simulink model "feed_fwd_2"  (Simulink 7.4)
settings: Solver=ode45  StartTime=0.0  StopTime=16e-6  MaxStep=1/(11*2140e6)  RelTol=1e-3
undefined symbols (not defined in the file): Fs, sided, Two
libraries: dsparch4 x10, dspsnks4 x3, simulink x1
settings Model: Creator=Dick  LastModifiedBy=Dick
settings DataIOCC: SignalLoggingName=sigsOut
settings OptimizationCC: BooleanDataType=off  InlineInvariantSignals=on  InitFltsAndDblsToZero=on
settings DebuggingCC: SaveWithParameterizedLinksMsg=none  SignalResolutionControl=TryResolveAllWithWarning  SolverPrmCheckMsg=none  MultiTaskDSMMsg=warning  MultiTaskCondExecSysMsg=none  StrictBusMsg=None
settings HardwareCC: TargetUnknown=on
settings RTWCC: IncludeERTFirstTime=on
settings GRTTargetCC: TargetFcnLib=ansi_tfl_tmw.mat

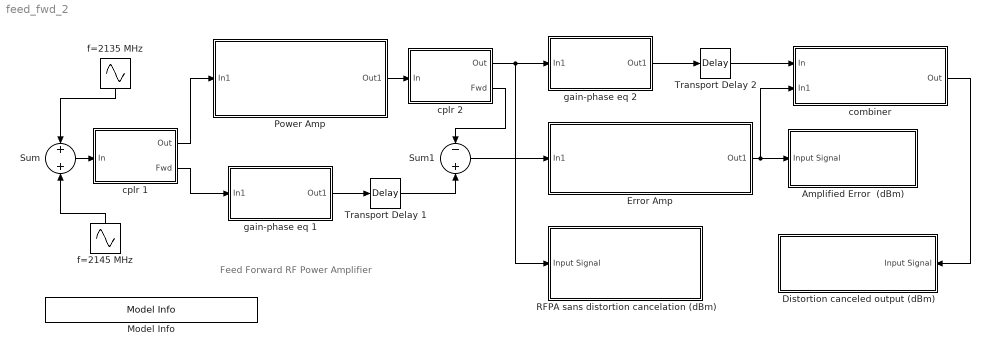
== system feed_fwd_2 ==
  note: Feed Forward RF Power Amplifier
  "  cplr 1" : Subsystem  mask{cplfac=-10}
      mask prompts: cplfac "Coupling Factor (in dB) ="
      mask Display: fprintf('Coupler  \n %5.2f dB', cplfac)
  "  cplr 2" : Subsystem  mask{cplfac=-6}
      mask prompts: cplfac "Coupling Factor (in dB) ="
      mask Display: disp(sprintf('Coupler  \n %5.2f dB', cplfac))
  Amplified Error  (dBm) : Subsystem  Description=Spectrum Analyzer  mask{BW=100e6, Fc=2140e6}
      mask prompts: BW "Bandwidth"; Fc "Center Freq"
      mask Display: fprintf('Spectrum Analyzer \n Fc=%7.2f MHz \n BW=%7.2f MHz',Fc/1e6,BW/1e6)
  Distortion canceled output (dBm) : Subsystem  Description=Spectrum Analyzer  mask{BW=100e6, Fc=2140e6}
      mask prompts: BW "Bandwidth"; Fc "Center Freq"
      mask Display: fprintf('Spectrum Analyzer \n Fc=%7.2f MHz \n BW=%7.2f MHz',Fc/1e6,BW/1e6)
  Error Amp : Subsystem  mask{dbg=12, Fc=2140, BW=100, Td=2}
      mask prompts: dbg "Gain in dB:"; Fc "Fcenter (MHz):"; BW "BW (MHz):"; Td "Time Delay (ns) :"
      mask Display:
      | fprintf(' Error Amp   Pg = %5.0f dB\n\n\n ',dbg);
      | fprintf(' Fcenter= %8.0f      BW= %5.0f MHz ', Fc, BW);
      | fprintf('\n\n\nTime Delay =%9.2f ns', Td);
  Model Info : simulink/Model-Wide Utilities/Model Info  SystemSampleTime=-1  InitialBlockCM=None  BlockCM=None  Frame=on  DisplayStringWithTags=Copywrite 2005-2010 The MathWorks, Inc.  HorizontalTextAlignment=Center  LeftAlignmentValue=0.5  SourceBlockDiagram=feed_fwd_2  TagMaxNumber=20
  Power Amp : Subsystem  mask{dbg=20, Fc=2140, BW=100, alpha=.02, Td=5}
      mask prompts: dbg "Gain in dB:"; Fc "Fcenter (MHz):"; BW "BW (MHz):"; alpha "Nonlinearity (0-1) :"; Td "Time Delay (ns) :"
      mask Display:
      | fprintf(' RFPA     Pg = %5.0f dB\n\n\n ',dbg);
      | fprintf('Fc= %6.0f    BW= %4.0fMHz ', Fc,BW);
      | fprintf('\n\n Nonlinearity =%9.4f', alpha);
      | fprintf('\n\n\n\n Time Delay =%9.2f ns', Td);
  RFPA sans distortion cancelation (dBm) : Subsystem  Description=Spectrum Analyzer  mask{BW=100e6, Fc=2140e6}
      mask prompts: BW "Bandwidth"; Fc "Center Freq"
      mask Display: fprintf('Spectrum Analyzer \n Fc=%7.2f MHz \n BW=%7.2f MHz',Fc/1e6,BW/1e6)
  Sum : Sum  OutDataType=sfix(16)  OutScaling=2^0  SaturateOnIntegerOverflow=on  InputSameDT=on  OutDataTypeStr=Inherit: Same as first input
  Sum1 : Sum  Inputs=-+  OutDataType=sfix(16)  OutScaling=2^0  SaturateOnIntegerOverflow=on  InputSameDT=on  OutDataTypeStr=Inherit: Same as first input
  Transport Delay 1 : TransportDelay  DelayTime=5e-9
  Transport Delay 2 : TransportDelay  DelayTime=2.0e-9
  combiner : Subsystem  mask{cplfac=-6}
      mask prompts: cplfac "Coupling Factor (in dB) ="
      mask Display: fprintf('Injection Coupler  \n %5.2f dB', cplfac)
  f=2135 MHz : Sin  Amplitude="((8e-3*50*10^(20/10))^0.5) /2    %  20 dBm"  Bias=0  Frequency=2*pi*(2140-5)*1e6;  Phase=0  Samples=10  SampleTime=0  Offset=0
  f=2145 MHz : Sin  Amplitude="((8e-3*50*10^(20/10))^0.5) /2    %  20 dBm"  Bias=0  Frequency=2*pi*(2140+5)*1e6  Phase=0  Samples=10  SampleTime=0  Offset=0
  gain-phase eq 1 : Subsystem
  gain-phase eq 2 : Subsystem
  wires:
  f=2135 MHz/1 -> Sum/1
  f=2145 MHz/1 -> Sum/2
  Sum/1 -> "  cplr 1"/1(In)
  "  cplr 1"/1(Out) -> Power Amp/1(In1)
  "  cplr 1"/2(Fwd) -> gain-phase eq 1/1(In1)
  gain-phase eq 1/1(Out1) -> Transport Delay 1/1
  Transport Delay 1/1 -> Sum1/2
  Sum1/1 -> Error Amp/1(In1)
  gain-phase eq 2/1(Out1) -> Transport Delay 2/1
  Transport Delay 2/1 -> combiner/1(In)
  Error Amp/1(Out1) -> combiner/2(In1), Amplified Error  (dBm)/1(Input Signal)
  combiner/1(Out) -> Distortion canceled output (dBm)/1(Input Signal)
  Power Amp/1(Out1) -> "  cplr 2"/1(In)
  "  cplr 2"/1(Out) -> gain-phase eq 2/1(In1), RFPA sans distortion cancelation (dBm)/1(Input Signal)
  "  cplr 2"/2(Fwd) -> Sum1/1

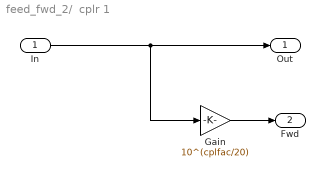
== system feed_fwd_2/  cplr 1 ==
  In : Inport  OutDataType=sfix(16)  OutScaling=2^0
  Gain : Gain  Gain=10^(cplfac/20)  ParameterDataType=sfix(16)  ParameterScaling=2^0  OutDataType=sfix(16)  OutScaling=2^0  SaturateOnIntegerOverflow=on  OutDataTypeStr=Inherit: Same as input  ParamDataTypeStr=Inherit: Same as input
  Out : Outport  OutDataType=sfix(16)  OutScaling=2^0
  Fwd : Outport  Port=2  OutDataType=sfix(16)  OutScaling=2^0
  wires:
  In/1 -> Out/1, Gain/1
  Gain/1 -> Fwd/1

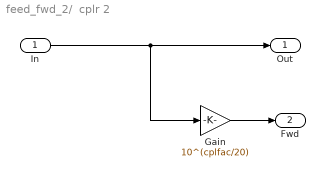
== system feed_fwd_2/  cplr 2 ==
  In : Inport  OutDataType=sfix(16)  OutScaling=2^0
  Gain : Gain  Gain=10^(cplfac/20)  ParameterDataType=sfix(16)  ParameterScaling=2^0  OutDataType=sfix(16)  OutScaling=2^0  SaturateOnIntegerOverflow=on  OutDataTypeStr=Inherit: Same as input  ParamDataTypeStr=Inherit: Same as input
  Out : Outport  OutDataType=sfix(16)  OutScaling=2^0
  Fwd : Outport  Port=2  OutDataType=sfix(16)  OutScaling=2^0
  wires:
  Gain/1 -> Fwd/1
  In/1 -> Gain/1, Out/1

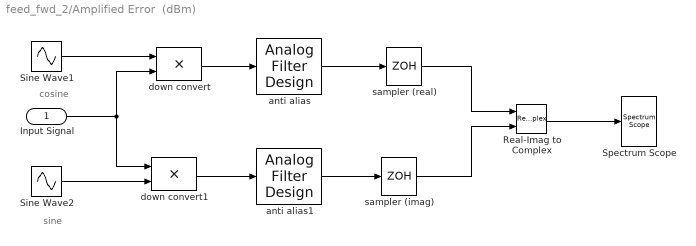
== system feed_fwd_2/Amplified Error  (dBm) ==
  note: sine
  note: cosine
  Input Signal : Inport  OutDataType=sfix(16)  OutScaling=2^0
  Real-Imag to Complex : RealImagToComplex
  Sine Wave1 : Sin  Amplitude=1/2  Bias=0  Frequency=2*pi*(Fc)  Phase=-pi/2  Samples=10  SampleTime=0  Offset=0
  Sine Wave2 : Sin  Amplitude=1/2  Bias=0  Frequency=2*pi*(Fc)  Phase=0  Samples=10  SampleTime=0  Offset=0
  Spectrum Scope : dspsnks4/Spectrum Scope  DialogController=dspdialog.SpectrumScope  DialogControllerArgs=DataTag0  SystemSampleTime=-1  ScopeProperties=off  Domain=Frequency  HorizSpan=1  UseBuffer=on  BufferSize=256  Overlap=64  inpFftLenInherit=off  FFTlength=128  numAvg=1  DisplayProperties=off  AxisGrid=on  Memory=off  FrameNumber=on  AxisLegend=off  AxisZoom=off  OpenScopeAtSimStart=on  OpenScopeImmediately=off  FigPos=[336 348 314 185]  AxisProperties=on  XUnits=Hertz  XRange=Two-sided ((-Fs/2...Fs/2])  XDisplay=0  InheritXIncr=on  XIncr=1.0  XLabel=Samples  XLimit=Auto  YUnits=dBm  XMax=1  XMin=0  YLabel=dBm  LineProperties=off  wintypeSpecScope=Hann  RsSpecScope=50  betaSpecScope=5  winsampSpecScope=Periodic  XAxisParamsVer=6.8
      settings: YMin=-50  YMax=50
  anti alias : dsparch4/Analog Filter Design  method=Elliptic  filttype=Lowpass  N=9  Wlo=BW*pi  Whi=80  Rp=1.2  Rs=100
  anti alias1 : dsparch4/Analog Filter Design  method=Elliptic  filttype=Lowpass  N=9  Wlo=BW*pi  Whi=80  Rp=1.2  Rs=100
  down convert : Product  OutDataType=sfix(16)  OutScaling=2^0  SaturateOnIntegerOverflow=on  InputSameDT=on  OutDataTypeStr=Inherit: Same as first input
  down convert1 : Product  OutDataType=sfix(16)  OutScaling=2^0  SaturateOnIntegerOverflow=on  InputSameDT=on  OutDataTypeStr=Inherit: Same as first input
  sampler (imag) : ZeroOrderHold  SampleTime=1/(1.28*BW)
  sampler (real) : ZeroOrderHold  SampleTime=1/(1.28*BW)
  wires:
  Real-Imag to Complex/1 -> Spectrum Scope/1
  sampler (imag)/1 -> Real-Imag to Complex/2
  sampler (real)/1 -> Real-Imag to Complex/1
  down convert1/1 -> anti alias1/1
  anti alias1/1 -> sampler (imag)/1
  Sine Wave2/1 -> down convert1/2
  Sine Wave1/1 -> down convert/1
  anti alias/1 -> sampler (real)/1
  down convert/1 -> anti alias/1
  Input Signal/1 -> down convert1/1, down convert/2

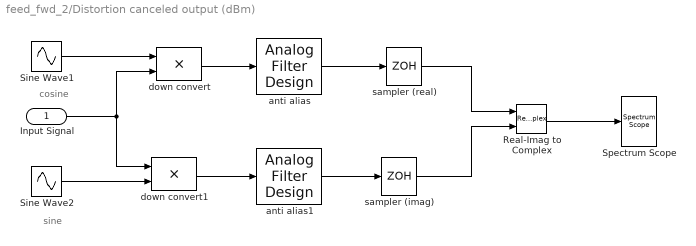
== system feed_fwd_2/Distortion canceled output (dBm) ==
  note: sine
  note: cosine
  Input Signal : Inport  OutDataType=sfix(16)  OutScaling=2^0
  Real-Imag to Complex : RealImagToComplex
  Sine Wave1 : Sin  Amplitude=1/2  Bias=0  Frequency=2*pi*(Fc)  Phase=-pi/2  Samples=10  SampleTime=0  Offset=0
  Sine Wave2 : Sin  Amplitude=1/2  Bias=0  Frequency=2*pi*(Fc)  Phase=0  Samples=10  SampleTime=0  Offset=0
  Spectrum Scope : dspsnks4/Spectrum Scope  DialogController=dspdialog.SpectrumScope  DialogControllerArgs=DataTag1  SystemSampleTime=-1  ScopeProperties=on  Domain=Frequency  HorizSpan=1  UseBuffer=on  BufferSize=256  Overlap=64  inpFftLenInherit=off  FFTlength=128  numAvg=2  DisplayProperties=off  AxisGrid=on  Memory=off  FrameNumber=on  AxisLegend=off  AxisZoom=off  OpenScopeAtSimStart=on  OpenScopeImmediately=off  FigPos=[663 351 289 183]  AxisProperties=off  XUnits=Hertz  XRange=Two-sided ((-Fs/2...Fs/2])  XDisplay=0  InheritXIncr=on  XIncr=1.0  XLabel=Samples  XLimit=Auto  YUnits=dBm  XMax=1  XMin=0  YLabel=dBm  LineProperties=off  wintypeSpecScope=Hann  RsSpecScope=50  betaSpecScope=5  winsampSpecScope=Periodic  XAxisParamsVer=6.8
      settings: YMin=-50  YMax=50
  anti alias : dsparch4/Analog Filter Design  method=Elliptic  filttype=Lowpass  N=9  Wlo=BW*pi  Whi=80  Rp=1.2  Rs=100
  anti alias1 : dsparch4/Analog Filter Design  method=Elliptic  filttype=Lowpass  N=9  Wlo=BW*pi  Whi=80  Rp=1.2  Rs=100
  down convert : Product  OutDataType=sfix(16)  OutScaling=2^0  SaturateOnIntegerOverflow=on  InputSameDT=on  OutDataTypeStr=Inherit: Same as first input
  down convert1 : Product  OutDataType=sfix(16)  OutScaling=2^0  SaturateOnIntegerOverflow=on  InputSameDT=on  OutDataTypeStr=Inherit: Same as first input
  sampler (imag) : ZeroOrderHold  SampleTime=1/(1.28*BW)
  sampler (real) : ZeroOrderHold  SampleTime=1/(1.28*BW)
  wires:
  Real-Imag to Complex/1 -> Spectrum Scope/1
  sampler (imag)/1 -> Real-Imag to Complex/2
  sampler (real)/1 -> Real-Imag to Complex/1
  down convert1/1 -> anti alias1/1
  anti alias1/1 -> sampler (imag)/1
  Sine Wave2/1 -> down convert1/2
  Sine Wave1/1 -> down convert/1
  anti alias/1 -> sampler (real)/1
  down convert/1 -> anti alias/1
  Input Signal/1 -> down convert1/1, down convert/2

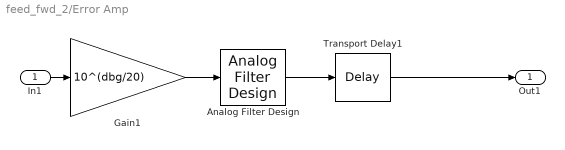
== system feed_fwd_2/Error Amp ==
  In1 : Inport  OutDataType=sfix(16)  OutScaling=2^0
  Analog Filter Design : dsparch4/Analog Filter Design  method=Elliptic  filttype=Bandpass  N=10  Wlo=2*pi*(Fc-BW/2)*1e6  Whi=2*pi*(Fc+BW/2)*1e6  Rp=2  Rs=40
  Gain1 : Gain  Gain=10^(dbg/20)  ParameterDataType=sfix(16)  ParameterScaling=2^0  OutDataType=sfix(16)  OutScaling=2^0  SaturateOnIntegerOverflow=on  OutDataTypeStr=Inherit: Same as input  ParamDataTypeStr=Inherit: Same as input
  Transport Delay1 : TransportDelay  DelayTime=Td*1e-9
  Out1 : Outport  OutDataType=sfix(16)  OutScaling=2^0
  wires:
  Analog Filter Design/1 -> Transport Delay1/1
  Gain1/1 -> Analog Filter Design/1
  In1/1 -> Gain1/1
  Transport Delay1/1 -> Out1/1

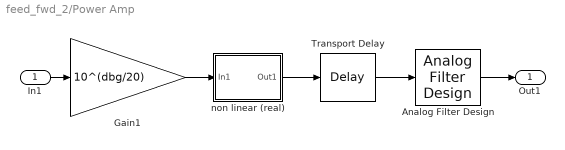
== system feed_fwd_2/Power Amp ==
  In1 : Inport  OutDataType=sfix(16)  OutScaling=2^0
  Analog Filter Design : dsparch4/Analog Filter Design  method=Elliptic  filttype=Bandpass  N=10  Wlo=2*pi*(Fc-BW/2)*1e6  Whi=2*pi*(Fc+BW/2)*1e6  Rp=2  Rs=40
  Gain1 : Gain  Gain=10^(dbg/20)  ParameterDataType=sfix(16)  ParameterScaling=2^0  OutDataType=sfix(16)  OutScaling=2^0  SaturateOnIntegerOverflow=on  OutDataTypeStr=Inherit: Same as input  ParamDataTypeStr=Inherit: Same as input
  Transport Delay : TransportDelay  DelayTime=Td*1e-9
  non linear (real) : Subsystem  mask{alpha=alpha}
      mask init:
      | x=-3:0.05:3;  y= (1/(alpha+eps))*tanh((alpha+eps)*x) ;
      mask Display: plot(x,y)
  Out1 : Outport  OutDataType=sfix(16)  OutScaling=2^0
  wires:
  In1/1 -> Gain1/1
  Gain1/1 -> non linear (real)/1(In1)
  non linear (real)/1(Out1) -> Transport Delay/1
  Analog Filter Design/1 -> Out1/1
  Transport Delay/1 -> Analog Filter Design/1

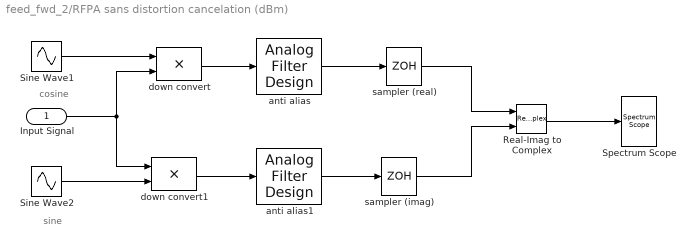
== system feed_fwd_2/RFPA sans distortion cancelation (dBm) ==
  note: cosine
  note: sine
  Input Signal : Inport  OutDataType=sfix(16)  OutScaling=2^0
  Real-Imag to Complex : RealImagToComplex
  Sine Wave1 : Sin  Amplitude=1/2  Bias=0  Frequency=2*pi*(Fc)  Phase=-pi/2  Samples=10  SampleTime=0  Offset=0
  Sine Wave2 : Sin  Amplitude=1/2  Bias=0  Frequency=2*pi*(Fc)  Phase=0  Samples=10  SampleTime=0  Offset=0
  Spectrum Scope : dspsnks4/Spectrum Scope  DialogController=dspdialog.SpectrumScope  DialogControllerArgs=DataTag2  SystemSampleTime=-1  ScopeProperties=off  Domain=Frequency  HorizSpan=1  UseBuffer=on  BufferSize=256  Overlap=64  inpFftLenInherit=off  FFTlength=128  numAvg=1  DisplayProperties=off  AxisGrid=on  Memory=off  FrameNumber=on  AxisLegend=off  AxisZoom=off  OpenScopeAtSimStart=on  OpenScopeImmediately=off  FigPos=[6 348 320 186]  AxisProperties=on  XUnits=Hertz  XRange=Two-sided ((-Fs/2...Fs/2])  XDisplay=0  InheritXIncr=on  XIncr=1.0  XLabel=Samples  XLimit=Auto  YUnits=dBm  XMax=1  XMin=0  YLabel=dBm  LineProperties=off  wintypeSpecScope=Hann  RsSpecScope=50  betaSpecScope=5  winsampSpecScope=Periodic  XAxisParamsVer=6.8
      settings: YMin=-50  YMax=50
  anti alias : dsparch4/Analog Filter Design  method=Elliptic  filttype=Lowpass  N=9  Wlo=BW*pi  Whi=80  Rp=1.2  Rs=100
  anti alias1 : dsparch4/Analog Filter Design  method=Elliptic  filttype=Lowpass  N=9  Wlo=BW*pi  Whi=80  Rp=1.2  Rs=100
  down convert : Product  OutDataType=sfix(16)  OutScaling=2^0  SaturateOnIntegerOverflow=on  InputSameDT=on  OutDataTypeStr=Inherit: Same as first input
  down convert1 : Product  OutDataType=sfix(16)  OutScaling=2^0  SaturateOnIntegerOverflow=on  InputSameDT=on  OutDataTypeStr=Inherit: Same as first input
  sampler (imag) : ZeroOrderHold  SampleTime=1/(1.28*BW)
  sampler (real) : ZeroOrderHold  SampleTime=1/(1.28*BW)
  wires:
  Input Signal/1 -> down convert/2, down convert1/1
  down convert/1 -> anti alias/1
  anti alias/1 -> sampler (real)/1
  Sine Wave1/1 -> down convert/1
  Sine Wave2/1 -> down convert1/2
  anti alias1/1 -> sampler (imag)/1
  down convert1/1 -> anti alias1/1
  sampler (real)/1 -> Real-Imag to Complex/1
  sampler (imag)/1 -> Real-Imag to Complex/2
  Real-Imag to Complex/1 -> Spectrum Scope/1

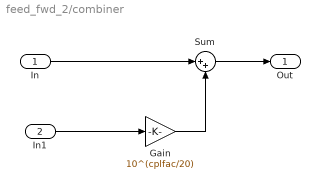
== system feed_fwd_2/combiner ==
  In : Inport  OutDataType=sfix(16)  OutScaling=2^0
  In1 : Inport  Port=2  OutDataType=sfix(16)  OutScaling=2^0
  Gain : Gain  Gain=10^(cplfac/20)  ParameterDataType=sfix(16)  ParameterScaling=2^0  OutDataType=sfix(16)  OutScaling=2^0  SaturateOnIntegerOverflow=on  OutDataTypeStr=Inherit: Same as input  ParamDataTypeStr=Inherit: Same as input
  Sum : Sum  Inputs=|++  OutDataType=sfix(16)  OutScaling=2^0  SaturateOnIntegerOverflow=on  InputSameDT=on  OutDataTypeStr=Inherit: Same as first input
  Out : Outport  OutDataType=sfix(16)  OutScaling=2^0
  wires:
  Gain/1 -> Sum/2
  Sum/1 -> Out/1
  In/1 -> Sum/1
  In1/1 -> Gain/1

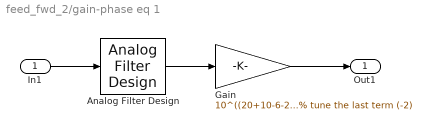
== system feed_fwd_2/gain-phase eq 1 ==
  In1 : Inport  OutDataType=sfix(16)  OutScaling=2^0
  Analog Filter Design : dsparch4/Analog Filter Design  method=Elliptic  filttype=Bandpass  N=10  Wlo=2*pi*(2140-50)*1e6  Whi=2*pi*(2140+50)*1e6  Rp=2  Rs=40
  Gain : Gain  Gain="10^((20+10-6-2)/20)  % tune the last term (-2)"  ParameterDataType=sfix(16)  ParameterScaling=2^0  OutDataType=sfix(16)  OutScaling=2^0  SaturateOnIntegerOverflow=on  OutDataTypeStr=Inherit: Same as input  ParamDataTypeStr=Inherit: Same as input
  Out1 : Outport  OutDataType=sfix(16)  OutScaling=2^0
  wires:
  In1/1 -> Analog Filter Design/1
  Analog Filter Design/1 -> Gain/1
  Gain/1 -> Out1/1

== system feed_fwd_2/gain-phase eq 2 ==
  In1 : Inport  OutDataType=sfix(16)  OutScaling=2^0
  Analog Filter Design : dsparch4/Analog Filter Design  method=Elliptic  filttype=Bandpass  N=10  Wlo=2*pi*(2140-50)*1e6  Whi=2*pi*(2140+50)*1e6  Rp=2  Rs=40
  Out1 : Outport  OutDataType=sfix(16)  OutScaling=2^0
  wires:
  Analog Filter Design/1 -> Out1/1
  In1/1 -> Analog Filter Design/1

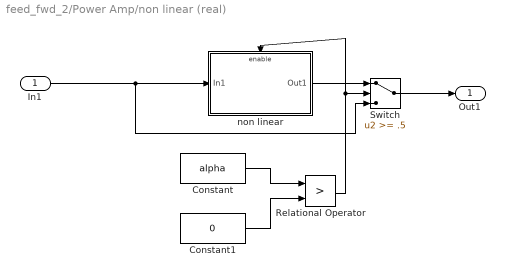
== system feed_fwd_2/Power Amp/non linear (real) ==
  In1 : Inport  OutDataType=sfix(16)  OutScaling=2^0
  Constant : Constant  Value=alpha  OutDataType=sfix(16)  OutScaling=2^0
  Constant1 : Constant  Value=0  OutDataType=sfix(16)  OutScaling=2^0
  Relational Operator : RelationalOperator  Operator=>  InputSameDT=on
  Switch : Switch  Threshold=.5  SaturateOnIntegerOverflow=on  InputSameDT=on
  "non linear " : Subsystem  TreatAsAtomicUnit=on
  Out1 : Outport  OutDataType=sfix(16)  OutScaling=2^0
  wires:
  In1/1 -> "non linear "/1(In1), Switch/3
  "non linear "/1(Out1) -> Switch/1
  Constant/1 -> Relational Operator/1
  Constant1/1 -> Relational Operator/2
  Relational Operator/1 -> Switch/2, "non linear "/Enable
  Switch/1 -> Out1/1

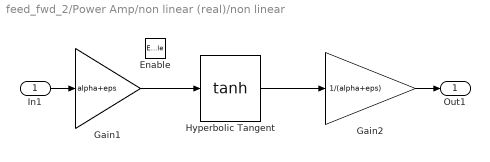
== system feed_fwd_2/Power Amp/non linear (real)/non linear  ==
  In1 : Inport  OutDataType=sfix(16)  OutScaling=2^0
  Enable : EnablePort
  Gain1 : Gain  Gain=alpha+eps  ParameterDataType=sfix(16)  ParameterScaling=2^0  OutDataType=sfix(16)  OutScaling=2^0  SaturateOnIntegerOverflow=on  OutDataTypeStr=Inherit: Same as input  ParamDataTypeStr=Inherit: Same as input
  Gain2 : Gain  Gain=1/(alpha+eps)  ParameterDataType=sfix(16)  ParameterScaling=2^0  OutDataType=sfix(16)  OutScaling=2^0  SaturateOnIntegerOverflow=on  OutDataTypeStr=Inherit: Same as input  ParamDataTypeStr=Inherit: Same as input
  Hyperbolic Tangent : Trigonometry  Operator=tanh
  Out1 : Outport  OutDataType=sfix(16)  OutScaling=2^0
  wires:
  Hyperbolic Tangent/1 -> Gain2/1
  Gain1/1 -> Hyperbolic Tangent/1
  Gain2/1 -> Out1/1
  In1/1 -> Gain1/1
